simulink model "SS_Model"  (R2015b)
settings: Solver=VariableStepAuto  StartTime=0.0  StopTime=10  RelTol=1e-3
undefined symbols (not defined in the file or in its folder): sys_cl, sys_cl_d
settings Model: Creator=Jcama  LastModifiedBy=Jcama

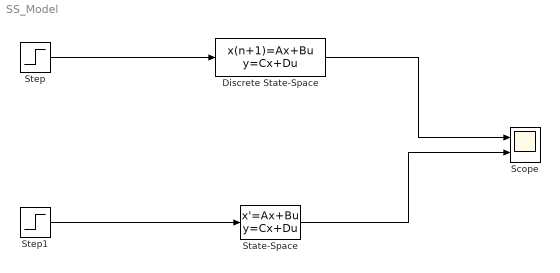
== system SS_Model ==
  Discrete State-Space : DiscreteStateSpace  A=sys_cl_d.a  B=sys_cl_d.b  C=sys_cl_d.c  D=sys_cl_d.d  SampleTime=0.1
  Scope : Scope  NumInputPorts=2
  State-Space : StateSpace  A=sys_cl.a  B=sys_cl.b  C=sys_cl.c  D=sys_cl.d  X0=0
  Step : Step  After=80  SampleTime=0.1
  Step1 : Step  After=80  SampleTime=0
  wires:
  Step/1 -> Discrete State-Space/1
  Discrete State-Space/1 -> Scope/1
  State-Space/1 -> Scope/2
  Step1/1 -> State-Space/1
